simulink model "sixDOF_model3"  (R2020b)
settings: Solver=VariableStepAuto  StartTime=0.0  StopTime=Inf  RelTol=1e-3
undefined symbols (not defined in the file or in its folder): X, Y, Z
libraries: sm_lib x31, nesl_utility x31
settings Model: EnablePacing=on  PacingRate=1.100000  Creator=Idrees  LastModifiedBy=brd
settings DataIOCC: ReturnWorkspaceOutputs=off
settings DebuggingCC: ArithmeticOperatorsInVariantConditions=warning
settings SFSimCC: CustomCodeUndefinedFunction=UseInterfaceOnly

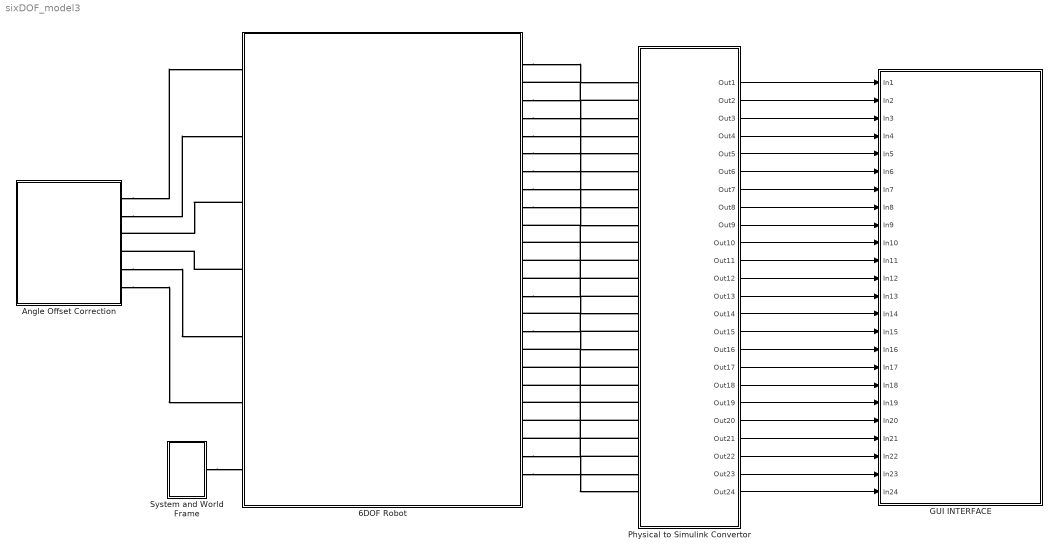
== system sixDOF_model3 ==
  6DOF Robot : Subsystem
  Angle Offset Correction : Subsystem
  GUI INTERFACE : Subsystem
  Physical to Simulink Convertor : Subsystem
  System and World Frame : Subsystem
  wires:
  Physical to Simulink Convertor/1(Out1) -> GUI INTERFACE/1(In1)
  Physical to Simulink Convertor/2(Out2) -> GUI INTERFACE/2(In2)
  Physical to Simulink Convertor/3(Out3) -> GUI INTERFACE/3(In3)
  Physical to Simulink Convertor/4(Out4) -> GUI INTERFACE/4(In4)
  Physical to Simulink Convertor/5(Out5) -> GUI INTERFACE/5(In5)
  Physical to Simulink Convertor/6(Out6) -> GUI INTERFACE/6(In6)
  Physical to Simulink Convertor/7(Out7) -> GUI INTERFACE/7(In7)
  Physical to Simulink Convertor/8(Out8) -> GUI INTERFACE/8(In8)
  Physical to Simulink Convertor/9(Out9) -> GUI INTERFACE/9(In9)
  Physical to Simulink Convertor/10(Out10) -> GUI INTERFACE/10(In10)
  Physical to Simulink Convertor/11(Out11) -> GUI INTERFACE/11(In11)
  Physical to Simulink Convertor/12(Out12) -> GUI INTERFACE/12(In12)
  Physical to Simulink Convertor/13(Out13) -> GUI INTERFACE/13(In13)
  Physical to Simulink Convertor/14(Out14) -> GUI INTERFACE/14(In14)
  Physical to Simulink Convertor/15(Out15) -> GUI INTERFACE/15(In15)
  Physical to Simulink Convertor/16(Out16) -> GUI INTERFACE/16(In16)
  Physical to Simulink Convertor/17(Out17) -> GUI INTERFACE/17(In17)
  Physical to Simulink Convertor/18(Out18) -> GUI INTERFACE/18(In18)
  Physical to Simulink Convertor/19(Out19) -> GUI INTERFACE/19(In19)
  Physical to Simulink Convertor/20(Out20) -> GUI INTERFACE/20(In20)
  Physical to Simulink Convertor/21(Out21) -> GUI INTERFACE/21(In21)
  Physical to Simulink Convertor/22(Out22) -> GUI INTERFACE/22(In22)
  Physical to Simulink Convertor/23(Out23) -> GUI INTERFACE/23(In23)
  Physical to Simulink Convertor/24(Out24) -> GUI INTERFACE/24(In24)
  connections:
  Angle Offset Correction/RConn1 -- 6DOF Robot/LConn1
  Angle Offset Correction/RConn2 -- 6DOF Robot/LConn2
  6DOF Robot/LConn3 -- Angle Offset Correction/RConn3
  6DOF Robot/LConn4 -- Angle Offset Correction/RConn4
  Angle Offset Correction/RConn5 -- 6DOF Robot/LConn5
  Angle Offset Correction/RConn6 -- 6DOF Robot/LConn6
  System and World Frame/RConn1 -- 6DOF Robot/LConn7
  6DOF Robot/RConn1 -- Physical to Simulink Convertor/LConn1
  Physical to Simulink Convertor/LConn2 -- 6DOF Robot/RConn2
  6DOF Robot/RConn3 -- Physical to Simulink Convertor/LConn3
  6DOF Robot/RConn4 -- Physical to Simulink Convertor/LConn4
  6DOF Robot/RConn5 -- Physical to Simulink Convertor/LConn5
  6DOF Robot/RConn6 -- Physical to Simulink Convertor/LConn6
  6DOF Robot/RConn7 -- Physical to Simulink Convertor/LConn7
  6DOF Robot/RConn8 -- Physical to Simulink Convertor/LConn8
  6DOF Robot/RConn9 -- Physical to Simulink Convertor/LConn9
  Physical to Simulink Convertor/LConn10 -- 6DOF Robot/RConn10
  Physical to Simulink Convertor/LConn11 -- 6DOF Robot/RConn11
  Physical to Simulink Convertor/LConn12 -- 6DOF Robot/RConn12
  Physical to Simulink Convertor/LConn13 -- 6DOF Robot/RConn13
  6DOF Robot/RConn14 -- Physical to Simulink Convertor/LConn14
  Physical to Simulink Convertor/LConn15 -- 6DOF Robot/RConn15
  6DOF Robot/RConn16 -- Physical to Simulink Convertor/LConn16
  Physical to Simulink Convertor/LConn17 -- 6DOF Robot/RConn17
  Physical to Simulink Convertor/LConn18 -- 6DOF Robot/RConn18
  Physical to Simulink Convertor/LConn19 -- 6DOF Robot/RConn19
  Physical to Simulink Convertor/LConn20 -- 6DOF Robot/RConn20
  Physical to Simulink Convertor/LConn21 -- 6DOF Robot/RConn21
  Physical to Simulink Convertor/LConn22 -- 6DOF Robot/RConn22
  6DOF Robot/RConn23 -- Physical to Simulink Convertor/LConn23
  6DOF Robot/RConn24 -- Physical to Simulink Convertor/LConn24

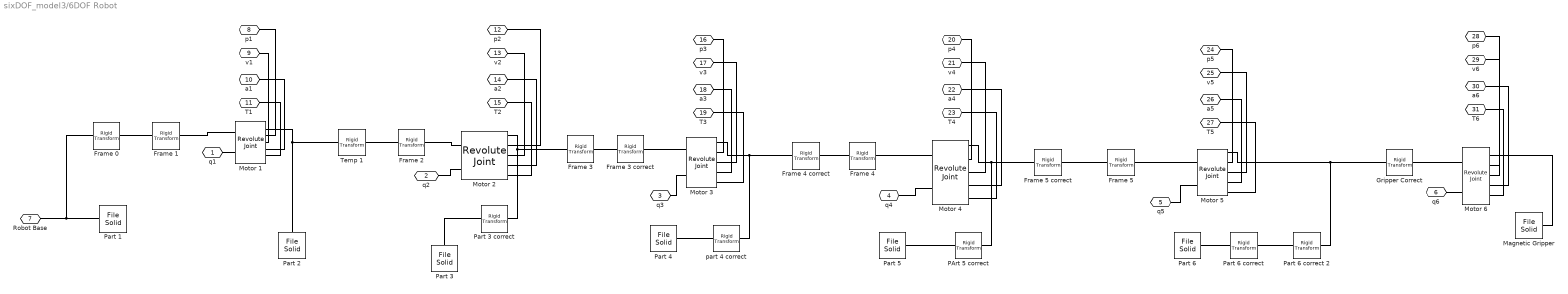
== system sixDOF_model3/6DOF Robot ==
  Frame 0 : sm_lib/Frames and Transforms/Rigid Transform  TranslationMethod=None  TranslationStandardOffset=0  TranslationLengthUnit=m  TranslationStandardAxis=+Z  TranslationCartesianOffset=[0 0 0]  TranslationROffset=0  TranslationROffsetUnits=m  TranslationZOffset=0  TranslationZOffsetUnits=m  TranslationThetaOffset=0  TranslationThetaOffsetUnits=deg  RotationMethod=StandardAxis  RotationAngleUnits=deg  RotationStandardAxis=+X  RotationAngle=90  RotationArbitraryAxis=[0 0 1]  FollAlignAxisA=+X  BaseAlignAxisA=+Y  FollAlignAxisB=+Y  BaseAlignAxisB=+Z  RotationSequenceAxes=FollowerAxes  RotationSequence=XYX  RotationSequenceAngles=[0 0 0]  RotationSequenceAnglesUnits=deg  RotationMatrix=[1 0 0; 0 1 0; 0 0 1]
  Frame 1 : sm_lib/Frames and Transforms/Rigid Transform  TranslationMethod=Cartesian  TranslationStandardOffset=60  TranslationLengthUnit=mm  TranslationStandardAxis=+Y  TranslationCartesianOffset=[0 60 0]  TranslationROffset=0  TranslationROffsetUnits=m  TranslationZOffset=0  TranslationZOffsetUnits=m  TranslationThetaOffset=0  TranslationThetaOffsetUnits=deg  RotationMethod=StandardAxis  RotationAngleUnits=deg  RotationStandardAxis=+X  RotationAngle=-90  RotationArbitraryAxis=[0 0 1]  FollAlignAxisA=+X  BaseAlignAxisA=+Y  FollAlignAxisB=+Y  BaseAlignAxisB=+Z  RotationSequenceAxes=FollowerAxes  RotationSequence=XYX  RotationSequenceAngles=[0 0 0]  RotationSequenceAnglesUnits=deg  RotationMatrix=[1 0 0; 0 1 0; 0 0 1]
  Frame 2 : sm_lib/Frames and Transforms/Rigid Transform  TranslationMethod=Cartesian  TranslationStandardOffset=0  TranslationLengthUnit=mm  TranslationStandardAxis=+Z  TranslationCartesianOffset=[0 26 29]  TranslationROffset=0  TranslationROffsetUnits=m  TranslationZOffset=0  TranslationZOffsetUnits=m  TranslationThetaOffset=0  TranslationThetaOffsetUnits=deg  RotationMethod=None  RotationAngleUnits=deg  RotationStandardAxis=+Z  RotationAngle=0.0  RotationArbitraryAxis=[0 0 1]  FollAlignAxisA=+X  BaseAlignAxisA=+Y  FollAlignAxisB=+Y  BaseAlignAxisB=+Z  RotationSequenceAxes=FollowerAxes  RotationSequence=XYX  RotationSequenceAngles=[0 0 0]  RotationSequenceAnglesUnits=deg  RotationMatrix=[1 0 0; 0 1 0; 0 0 1]
  Frame 3 : sm_lib/Frames and Transforms/Rigid Transform  TranslationMethod=Cartesian  TranslationStandardOffset=0  TranslationLengthUnit=mm  TranslationStandardAxis=+Z  TranslationCartesianOffset=[210 0 17]  TranslationROffset=0  TranslationROffsetUnits=m  TranslationZOffset=0  TranslationZOffsetUnits=m  TranslationThetaOffset=0  TranslationThetaOffsetUnits=deg  RotationMethod=StandardAxis  RotationAngleUnits=deg  RotationStandardAxis=+Z  RotationAngle=90  RotationArbitraryAxis=[0 0 1]  FollAlignAxisA=+X  BaseAlignAxisA=+Y  FollAlignAxisB=+Y  BaseAlignAxisB=+Z  RotationSequenceAxes=FollowerAxes  RotationSequence=XYX  RotationSequenceAngles=[0 0 0]  RotationSequenceAnglesUnits=deg  RotationMatrix=[1 0 0; 0 1 0; 0 0 1]
  Frame 3 correct : sm_lib/Frames and Transforms/Rigid Transform  TranslationMethod=Cartesian  TranslationStandardOffset=0  TranslationLengthUnit=mm  TranslationStandardAxis=+Z  TranslationCartesianOffset=[0 0 -60]  TranslationROffset=0  TranslationROffsetUnits=m  TranslationZOffset=0  TranslationZOffsetUnits=m  TranslationThetaOffset=0  TranslationThetaOffsetUnits=deg  RotationMethod=None  RotationAngleUnits=deg  RotationStandardAxis=+Z  RotationAngle=0.0  RotationArbitraryAxis=[0 0 1]  FollAlignAxisA=+X  BaseAlignAxisA=+Y  FollAlignAxisB=+Y  BaseAlignAxisB=+Z  RotationSequenceAxes=FollowerAxes  RotationSequence=XYX  RotationSequenceAngles=[0 0 0]  RotationSequenceAnglesUnits=deg  RotationMatrix=[1 0 0; 0 1 0; 0 0 1]
  Frame 4 : sm_lib/Frames and Transforms/Rigid Transform  TranslationMethod=Cartesian  TranslationStandardOffset=0  TranslationLengthUnit=mm  TranslationStandardAxis=+Z  TranslationCartesianOffset=[0 0 80]  TranslationROffset=0  TranslationROffsetUnits=m  TranslationZOffset=0  TranslationZOffsetUnits=m  TranslationThetaOffset=0  TranslationThetaOffsetUnits=deg  RotationMethod=StandardAxis  RotationAngleUnits=deg  RotationStandardAxis=+Z  RotationAngle=180  RotationArbitraryAxis=[0 0 1]  FollAlignAxisA=+X  BaseAlignAxisA=+Y  FollAlignAxisB=+Y  BaseAlignAxisB=+Z  RotationSequenceAxes=FollowerAxes  RotationSequence=XYX  RotationSequenceAngles=[0 0 0]  RotationSequenceAnglesUnits=deg  RotationMatrix=[1 0 0; 0 1 0; 0 0 1]
  Frame 4 correct : sm_lib/Frames and Transforms/Rigid Transform  TranslationMethod=Cartesian  TranslationStandardOffset=0  TranslationLengthUnit=mm  TranslationStandardAxis=+Z  TranslationCartesianOffset=[-180 0 0]  TranslationROffset=0  TranslationROffsetUnits=m  TranslationZOffset=0  TranslationZOffsetUnits=m  TranslationThetaOffset=0  TranslationThetaOffsetUnits=deg  RotationMethod=None  RotationAngleUnits=deg  RotationStandardAxis=+Z  RotationAngle=0.0  RotationArbitraryAxis=[0 0 1]  FollAlignAxisA=+X  BaseAlignAxisA=+Y  FollAlignAxisB=+Y  BaseAlignAxisB=+Z  RotationSequenceAxes=FollowerAxes  RotationSequence=XYX  RotationSequenceAngles=[0 0 0]  RotationSequenceAnglesUnits=deg  RotationMatrix=[1 0 0; 0 1 0; 0 0 1]
  "Frame 5 " : sm_lib/Frames and Transforms/Rigid Transform  TranslationMethod=Cartesian  TranslationStandardOffset=0  TranslationLengthUnit=mm  TranslationStandardAxis=+Z  TranslationCartesianOffset=[0 0 44.5]  TranslationROffset=0  TranslationROffsetUnits=m  TranslationZOffset=0  TranslationZOffsetUnits=m  TranslationThetaOffset=0  TranslationThetaOffsetUnits=deg  RotationMethod=None  RotationAngleUnits=deg  RotationStandardAxis=+Z  RotationAngle=0.0  RotationArbitraryAxis=[0 0 1]  FollAlignAxisA=+X  BaseAlignAxisA=+Y  FollAlignAxisB=+Y  BaseAlignAxisB=+Z  RotationSequenceAxes=FollowerAxes  RotationSequence=XYX  RotationSequenceAngles=[0 0 0]  RotationSequenceAnglesUnits=deg  RotationMatrix=[1 0 0; 0 1 0; 0 0 1]
  Frame 5 correct : sm_lib/Frames and Transforms/Rigid Transform  TranslationMethod=Cartesian  TranslationStandardOffset=0  TranslationLengthUnit=mm  TranslationStandardAxis=+Z  TranslationCartesianOffset=[0 0 21]  TranslationROffset=0  TranslationROffsetUnits=m  TranslationZOffset=0  TranslationZOffsetUnits=m  TranslationThetaOffset=0  TranslationThetaOffsetUnits=deg  RotationMethod=RotationSequence  RotationAngleUnits=deg  RotationStandardAxis=+X  RotationAngle=90  RotationArbitraryAxis=[0 0 1]  FollAlignAxisA=+X  BaseAlignAxisA=+Y  FollAlignAxisB=+Y  BaseAlignAxisB=+Z  RotationSequenceAxes=FollowerAxes  RotationSequence=XZY  RotationSequenceAngles=[90 90 0]  RotationSequenceAnglesUnits=deg  RotationMatrix=[1 0 0; 0 1 0; 0 0 1]
  Gripper Correct : sm_lib/Frames and Transforms/Rigid Transform  TranslationMethod=Cartesian  TranslationStandardOffset=0  TranslationLengthUnit=mm  TranslationStandardAxis=+Z  TranslationCartesianOffset=[-15 0 0]  TranslationROffset=0  TranslationROffsetUnits=m  TranslationZOffset=0  TranslationZOffsetUnits=m  TranslationThetaOffset=0  TranslationThetaOffsetUnits=deg  RotationMethod=StandardAxis  RotationAngleUnits=deg  RotationStandardAxis=+Y  RotationAngle=-90  RotationArbitraryAxis=[0 0 1]  FollAlignAxisA=+X  BaseAlignAxisA=+Y  FollAlignAxisB=+Y  BaseAlignAxisB=+Z  RotationSequenceAxes=FollowerAxes  RotationSequence=XYX  RotationSequenceAngles=[0 0 0]  RotationSequenceAnglesUnits=deg  RotationMatrix=[1 0 0; 0 1 0; 0 0 1]
  Magnetic Gripper : sm_lib/Body Elements/File Solid  ExtGeomFileName=/home/brd/Dropbox/School/senior-design/src/matlab/6DOF_Robot/Part7_MagneticGripper2.STEP  UnitType=FromFile  ExtGeomFileUnits=m  StepReaderType=OCC  ExportConvexHullGeometry=off  InertiaType=CalculateFromGeometry  Mass=1  MassUnits=kg  CenterOfMass=[0 0 0]  CenterOfMassUnits=m  MomentsOfInertia=[1 1 1]  MomentsOfInertiaUnits=kg*m^2  ProductsOfInertia=[0 0 0]  ProductsOfInertiaUnits=kg*m^2  BasedOnType=Density  Density=1240  DensityUnits=kg/m^3  DoExposeReferenceFrame=on  SerializedFrames=<Frames/>  GraphicType=FromGeometry  MarkerShape=Sphere  MarkerSize=10  GraphicVisPropType=SimpleVisualProperties  GraphicDiffuseColor=[0.2 0.2 0.2]  GraphicSpecularColor=[0.5 0.5 0.5 1.0]  GraphicAmbientColor=[0.15 0.15 0.15 1.0]  GraphicEmissiveColor=[0.0 0.0 0.0 1.0]  GraphicShininess=75  GraphicOpacity=1.0
  Motor {1..6} (6 alike) : sm_lib/Joints/Revolute Joint  JointMode=Normal  SenseConstraintForce=off  SenseConstraintForceX=off  SenseConstraintForceY=off  SenseConstraintForceZ=off  SenseConstraintTorque=off  SenseConstraintTorqueX=off  SenseConstraintTorqueY=off  SenseConstraintTorqueZ=off  SenseTotalForce=off  SenseTotalForceX=off  SenseTotalForceY=off  SenseTotalForceZ=off  SenseTotalTorque=off  SenseTotalTorqueX=off  SenseTotalTorqueY=off  SenseTotalTorqueZ=off  CompositeWrenchDir=FollowerOnBase  CompositeWrenchFrame=BaseFrame  EquilibriumPosition=0  EquilibriumPositionUnits=deg  SpringStiffness=0  SpringStiffnessUnits=N*m/deg  DampingCoefficient=0  DampingCoefficientUnits=N*m/(deg/s)  TorqueActuationMode=ComputedTorque  MotionActuationMode=InputMotion  SensePosition=on  SenseVelocity=on  SenseAcceleration=on  SenseTorqueForce=on  SenseLowerLimitTorqueForce=off  SenseUpperLimitTorqueForce=off  LowerLimitSpecify=off  LowerLimitBound=-90  LowerLimitBoundUnits=deg  LowerLimitStiffness=1e4  LowerLimitStiffnessUnits=N*m/deg  LowerLimitDamping=10  LowerLimitDampingUnits=N*m/(deg/s)  LowerLimitTransitionRegionWidth=0.1  LowerLimitTransitionRegionWidthUnits=deg  UpperLimitSpecify=off  UpperLimitBound=90  UpperLimitBoundUnits=deg  UpperLimitStiffness=1e4  UpperLimitStiffnessUnits=N*m/deg  UpperLimitDamping=10  UpperLimitDampingUnits=N*m/(deg/s)  UpperLimitTransitionRegionWidth=0.1  UpperLimitTransitionRegionWidthUnits=deg  PositionTargetSpecify=off  PositionTargetPriority=High  PositionTargetValue=0  PositionTargetValueUnits=deg  VelocityTargetSpecify=off  VelocityTargetPriority=High  VelocityTargetValue=0  VelocityTargetValueUnits=deg/s
  PArt 5 correct : sm_lib/Frames and Transforms/Rigid Transform  TranslationMethod=None  TranslationStandardOffset=0  TranslationLengthUnit=m  TranslationStandardAxis=+Z  TranslationCartesianOffset=[0 0 0]  TranslationROffset=0  TranslationROffsetUnits=m  TranslationZOffset=0  TranslationZOffsetUnits=m  TranslationThetaOffset=0  TranslationThetaOffsetUnits=deg  RotationMethod=StandardAxis  RotationAngleUnits=deg  RotationStandardAxis=+X  RotationAngle=180  RotationArbitraryAxis=[0 0 1]  FollAlignAxisA=+X  BaseAlignAxisA=+Y  FollAlignAxisB=+Y  BaseAlignAxisB=+Z  RotationSequenceAxes=FollowerAxes  RotationSequence=XYX  RotationSequenceAngles=[0 0 0]  RotationSequenceAnglesUnits=deg  RotationMatrix=[1 0 0; 0 1 0; 0 0 1]
  "Part 1 " : sm_lib/Body Elements/File Solid  ExtGeomFileName=/home/brd/Dropbox/School/senior-design/src/matlab/6DOF_Robot/Part1.STEP  UnitType=FromFile  ExtGeomFileUnits=m  StepReaderType=OCC  ExportConvexHullGeometry=off  InertiaType=CalculateFromGeometry  Mass=1  MassUnits=kg  CenterOfMass=[0 0 0]  CenterOfMassUnits=m  MomentsOfInertia=[1 1 1]  MomentsOfInertiaUnits=kg*m^2  ProductsOfInertia=[0 0 0]  ProductsOfInertiaUnits=kg*m^2  BasedOnType=Density  Density=1240  DensityUnits=kg/m^3  DoExposeReferenceFrame=on  SerializedFrames=<Frames/>  GraphicType=FromGeometry  MarkerShape=Sphere  MarkerSize=10  GraphicVisPropType=SimpleVisualProperties  GraphicDiffuseColor=[1.0 0.6 0.2]  GraphicSpecularColor=[0.5 0.5 0.5 1.0]  GraphicAmbientColor=[0.15 0.15 0.15 1.0]  GraphicEmissiveColor=[0.0 0.0 0.0 1.0]  GraphicShininess=75  GraphicOpacity=1.0
  Part 2 : sm_lib/Body Elements/File Solid  ExtGeomFileName=/home/brd/Dropbox/School/senior-design/src/matlab/6DOF_Robot/Part2.STEP  UnitType=FromFile  ExtGeomFileUnits=m  StepReaderType=OCC  ExportConvexHullGeometry=off  InertiaType=CalculateFromGeometry  Mass=1  MassUnits=kg  CenterOfMass=[0 0 0]  CenterOfMassUnits=m  MomentsOfInertia=[1 1 1]  MomentsOfInertiaUnits=kg*m^2  ProductsOfInertia=[0 0 0]  ProductsOfInertiaUnits=kg*m^2  BasedOnType=Density  Density=1240  DensityUnits=kg/m^3  DoExposeReferenceFrame=on  SerializedFrames=<Frames/>  GraphicType=FromGeometry  MarkerShape=Sphere  MarkerSize=10  GraphicVisPropType=SimpleVisualProperties  GraphicDiffuseColor=[1.0 0.4 0.0]  GraphicSpecularColor=[0.5 0.5 0.5 1.0]  GraphicAmbientColor=[0.15 0.15 0.15 1.0]  GraphicEmissiveColor=[0.0 0.0 0.0 1.0]  GraphicShininess=75  GraphicOpacity=1.0
  Part 3 : sm_lib/Body Elements/File Solid  ExtGeomFileName=/home/brd/Dropbox/School/senior-design/src/matlab/6DOF_Robot/Part3.STEP  UnitType=FromFile  ExtGeomFileUnits=m  StepReaderType=OCC  ExportConvexHullGeometry=off  InertiaType=CalculateFromGeometry  Mass=1  MassUnits=kg  CenterOfMass=[0 0 0]  CenterOfMassUnits=m  MomentsOfInertia=[1 1 1]  MomentsOfInertiaUnits=kg*m^2  ProductsOfInertia=[0 0 0]  ProductsOfInertiaUnits=kg*m^2  BasedOnType=Density  Density=1240  DensityUnits=kg/m^3  DoExposeReferenceFrame=on  SerializedFrames=<Frames/>  GraphicType=FromGeometry  MarkerShape=Sphere  MarkerSize=10  GraphicVisPropType=SimpleVisualProperties  GraphicDiffuseColor=[1.0 0.4 0.0]  GraphicSpecularColor=[0.5 0.5 0.5 1.0]  GraphicAmbientColor=[0.15 0.15 0.15 1.0]  GraphicEmissiveColor=[0.0 0.0 0.0 1.0]  GraphicShininess=75  GraphicOpacity=1.0
  Part 3 correct : sm_lib/Frames and Transforms/Rigid Transform  TranslationMethod=Cartesian  TranslationStandardOffset=0  TranslationLengthUnit=mm  TranslationStandardAxis=+Z  TranslationCartesianOffset=[-210/2 0 0]  TranslationROffset=0  TranslationROffsetUnits=m  TranslationZOffset=0  TranslationZOffsetUnits=m  TranslationThetaOffset=0  TranslationThetaOffsetUnits=deg  RotationMethod=None  RotationAngleUnits=deg  RotationStandardAxis=+Z  RotationAngle=0.0  RotationArbitraryAxis=[0 0 1]  FollAlignAxisA=+X  BaseAlignAxisA=+Y  FollAlignAxisB=+Y  BaseAlignAxisB=+Z  RotationSequenceAxes=FollowerAxes  RotationSequence=XYX  RotationSequenceAngles=[0 0 0]  RotationSequenceAnglesUnits=deg  RotationMatrix=[1 0 0; 0 1 0; 0 0 1]
  Part 4 : sm_lib/Body Elements/File Solid  ExtGeomFileName=/home/brd/Dropbox/School/senior-design/src/matlab/6DOF_Robot/Part4.STEP  UnitType=FromFile  ExtGeomFileUnits=m  StepReaderType=OCC  ExportConvexHullGeometry=off  InertiaType=CalculateFromGeometry  Mass=1  MassUnits=kg  CenterOfMass=[0 0 0]  CenterOfMassUnits=m  MomentsOfInertia=[1 1 1]  MomentsOfInertiaUnits=kg*m^2  ProductsOfInertia=[0 0 0]  ProductsOfInertiaUnits=kg*m^2  BasedOnType=Density  Density=1240  DensityUnits=kg/m^3  DoExposeReferenceFrame=on  SerializedFrames=<Frames/>  GraphicType=FromGeometry  MarkerShape=Sphere  MarkerSize=10  GraphicVisPropType=SimpleVisualProperties  GraphicDiffuseColor=[1.0 0.4 0.0]  GraphicSpecularColor=[0.5 0.5 0.5 1.0]  GraphicAmbientColor=[0.15 0.15 0.15 1.0]  GraphicEmissiveColor=[0.0 0.0 0.0 1.0]  GraphicShininess=75  GraphicOpacity=1.0
  Part 5 : sm_lib/Body Elements/File Solid  ExtGeomFileName=/home/brd/Dropbox/School/senior-design/src/matlab/6DOF_Robot/Part5.STEP  UnitType=FromFile  ExtGeomFileUnits=m  StepReaderType=OCC  ExportConvexHullGeometry=off  InertiaType=CalculateFromGeometry  Mass=1  MassUnits=kg  CenterOfMass=[0 0 0]  CenterOfMassUnits=m  MomentsOfInertia=[1 1 1]  MomentsOfInertiaUnits=kg*m^2  ProductsOfInertia=[0 0 0]  ProductsOfInertiaUnits=kg*m^2  BasedOnType=Density  Density=1240  DensityUnits=kg/m^3  DoExposeReferenceFrame=on  SerializedFrames=<Frames/>  GraphicType=FromGeometry  MarkerShape=Sphere  MarkerSize=10  GraphicVisPropType=SimpleVisualProperties  GraphicDiffuseColor=[1.0 0.4 0.0]  GraphicSpecularColor=[0.5 0.5 0.5 1.0]  GraphicAmbientColor=[0.15 0.15 0.15 1.0]  GraphicEmissiveColor=[0.0 0.0 0.0 1.0]  GraphicShininess=75  GraphicOpacity=1.0
  Part 6 : sm_lib/Body Elements/File Solid  ExtGeomFileName=/home/brd/Dropbox/School/senior-design/src/matlab/6DOF_Robot/Part6.STEP  UnitType=FromFile  ExtGeomFileUnits=m  StepReaderType=OCC  ExportConvexHullGeometry=off  InertiaType=CalculateFromGeometry  Mass=1  MassUnits=kg  CenterOfMass=[0 0 0]  CenterOfMassUnits=m  MomentsOfInertia=[1 1 1]  MomentsOfInertiaUnits=kg*m^2  ProductsOfInertia=[0 0 0]  ProductsOfInertiaUnits=kg*m^2  BasedOnType=Density  Density=1240  DensityUnits=kg/m^3  DoExposeReferenceFrame=on  SerializedFrames=<Frames/>  GraphicType=FromGeometry  MarkerShape=Sphere  MarkerSize=10  GraphicVisPropType=SimpleVisualProperties  GraphicDiffuseColor=[1.0 0.4 0.0]  GraphicSpecularColor=[0.5 0.5 0.5 1.0]  GraphicAmbientColor=[0.15 0.15 0.15 1.0]  GraphicEmissiveColor=[0.0 0.0 0.0 1.0]  GraphicShininess=75  GraphicOpacity=1.0
  Part 6 correct : sm_lib/Frames and Transforms/Rigid Transform  TranslationMethod=Cartesian  TranslationStandardOffset=0  TranslationLengthUnit=mm  TranslationStandardAxis=+Z  TranslationCartesianOffset=[0 0 15]  TranslationROffset=0  TranslationROffsetUnits=m  TranslationZOffset=0  TranslationZOffsetUnits=m  TranslationThetaOffset=0  TranslationThetaOffsetUnits=deg  RotationMethod=None  RotationAngleUnits=deg  RotationStandardAxis=+X  RotationAngle=90  RotationArbitraryAxis=[0 0 1]  FollAlignAxisA=+X  BaseAlignAxisA=+Y  FollAlignAxisB=+Y  BaseAlignAxisB=+Z  RotationSequenceAxes=FollowerAxes  RotationSequence=XYX  RotationSequenceAngles=[0 0 0]  RotationSequenceAnglesUnits=deg  RotationMatrix=[1 0 0; 0 1 0; 0 0 1]
  Part 6 correct 2 : sm_lib/Frames and Transforms/Rigid Transform  TranslationMethod=None  TranslationStandardOffset=0  TranslationLengthUnit=m  TranslationStandardAxis=+Z  TranslationCartesianOffset=[0 0 0]  TranslationROffset=0  TranslationROffsetUnits=m  TranslationZOffset=0  TranslationZOffsetUnits=m  TranslationThetaOffset=0  TranslationThetaOffsetUnits=deg  RotationMethod=RotationSequence  RotationAngleUnits=deg  RotationStandardAxis=+Z  RotationAngle=0.0  RotationArbitraryAxis=[0 0 1]  FollAlignAxisA=+X  BaseAlignAxisA=+Y  FollAlignAxisB=+Y  BaseAlignAxisB=+Z  RotationSequenceAxes=FollowerAxes  RotationSequence=ZYX  RotationSequenceAngles=[90 -90 0]  RotationSequenceAnglesUnits=deg  RotationMatrix=[1 0 0; 0 1 0; 0 0 1]
  Temp 1 : sm_lib/Frames and Transforms/Rigid Transform  TranslationMethod=None  TranslationStandardOffset=0  TranslationLengthUnit=m  TranslationStandardAxis=+Z  TranslationCartesianOffset=[0 0 0]  TranslationROffset=0  TranslationROffsetUnits=m  TranslationZOffset=0  TranslationZOffsetUnits=m  TranslationThetaOffset=0  TranslationThetaOffsetUnits=deg  RotationMethod=StandardAxis  RotationAngleUnits=deg  RotationStandardAxis=+X  RotationAngle=90  RotationArbitraryAxis=[0 0 1]  FollAlignAxisA=+X  BaseAlignAxisA=+Y  FollAlignAxisB=+Y  BaseAlignAxisB=+Z  RotationSequenceAxes=FollowerAxes  RotationSequence=XYX  RotationSequenceAngles=[0 0 0]  RotationSequenceAnglesUnits=deg  RotationMatrix=[1 0 0; 0 1 0; 0 0 1]
  part 4 correct : sm_lib/Frames and Transforms/Rigid Transform  TranslationMethod=Cartesian  TranslationStandardOffset=0  TranslationLengthUnit=mm  TranslationStandardAxis=+Z  TranslationCartesianOffset=[180/2 0 0]  TranslationROffset=0  TranslationROffsetUnits=m  TranslationZOffset=0  TranslationZOffsetUnits=m  TranslationThetaOffset=0  TranslationThetaOffsetUnits=deg  RotationMethod=None  RotationAngleUnits=deg  RotationStandardAxis=+Z  RotationAngle=0.0  RotationArbitraryAxis=[0 0 1]  FollAlignAxisA=+X  BaseAlignAxisA=+Y  FollAlignAxisB=+Y  BaseAlignAxisB=+Z  RotationSequenceAxes=FollowerAxes  RotationSequence=XYX  RotationSequenceAngles=[0 0 0]  RotationSequenceAnglesUnits=deg  RotationMatrix=[1 0 0; 0 1 0; 0 0 1]
  q1 : PMIOPort  Side=Left
  q2 : PMIOPort  Port=2  Side=Left
  q3 : PMIOPort  Port=3  Side=Left
  q4 : PMIOPort  Port=4  Side=Left
  q5 : PMIOPort  Port=5  Side=Left
  q6 : PMIOPort  Port=6  Side=Left
  Robot Base : PMIOPort  Port=7  Side=Left
  p1 : PMIOPort  Port=8  Side=Right
  v1 : PMIOPort  Port=9  Side=Right
  a1 : PMIOPort  Port=10  Side=Right
  T1 : PMIOPort  Port=11  Side=Right
  p2 : PMIOPort  Port=12  Side=Right
  v2 : PMIOPort  Port=13  Side=Right
  a2 : PMIOPort  Port=14  Side=Right
  T2 : PMIOPort  Port=15  Side=Right
  p3 : PMIOPort  Port=16  Side=Right
  v3 : PMIOPort  Port=17  Side=Right
  a3 : PMIOPort  Port=18  Side=Right
  T3 : PMIOPort  Port=19  Side=Right
  p4 : PMIOPort  Port=20  Side=Right
  v4 : PMIOPort  Port=21  Side=Right
  a4 : PMIOPort  Port=22  Side=Right
  T4 : PMIOPort  Port=23  Side=Right
  p5 : PMIOPort  Port=24  Side=Right
  v5 : PMIOPort  Port=25  Side=Right
  a5 : PMIOPort  Port=26  Side=Right
  T5 : PMIOPort  Port=27  Side=Right
  p6 : PMIOPort  Port=28  Side=Right
  v6 : PMIOPort  Port=29  Side=Right
  a6 : PMIOPort  Port=30  Side=Right
  T6 : PMIOPort  Port=31  Side=Right
  connections:
  Motor 1/LConn1 -- Frame 1/RConn1
  Motor 4/RConn1 -- Frame 5 correct/LConn1 -- PArt 5 correct/RConn1
  part 4 correct/RConn1 -- Motor 3/RConn1 -- Frame 4 correct/LConn1
  Frame 1/LConn1 -- Frame 0/RConn1
  Part 6 correct/LConn1 -- Part 6/RConn1
  part 4 correct/LConn1 -- Part 4/RConn1
  Magnetic Gripper/RConn1 -- Motor 6/RConn1
  Frame 4/LConn1 -- Frame 4 correct/RConn1
  "Part 1 "/RConn1 -- Robot Base/RConn1 -- Frame 0/LConn1
  Motor 1/RConn1 -- Temp 1/LConn1 -- Part 2/RConn1
  Part 6 correct 2/RConn1 -- Motor 5/RConn1 -- Gripper Correct/LConn1
  Motor 6/LConn1 -- Gripper Correct/RConn1
  Frame 3 correct/LConn1 -- Frame 3/RConn1
  Temp 1/RConn1 -- Frame 2/LConn1
  Motor 3/LConn1 -- Frame 3 correct/RConn1
  Motor 2/LConn2 -- q2/RConn1
  "Frame 5 "/LConn1 -- Frame 5 correct/RConn1
  Motor 2/RConn1 -- Part 3 correct/RConn1 -- Frame 3/LConn1
  Motor 2/LConn1 -- Frame 2/RConn1
  Part 3 correct/LConn1 -- Part 3/RConn1
  Frame 4/RConn1 -- Motor 4/LConn1
  Motor 5/LConn1 -- "Frame 5 "/RConn1
  PArt 5 correct/LConn1 -- Part 5/RConn1
  Part 6 correct 2/LConn1 -- Part 6 correct/RConn1
  Motor 1/LConn2 -- q1/RConn1
  Motor 3/LConn2 -- q3/RConn1
  Motor 4/LConn2 -- q4/RConn1
  Motor 5/LConn2 -- q5/RConn1
  q6/RConn1 -- Motor 6/LConn2
  T2/RConn1 -- Motor 2/RConn5
  p2/RConn1 -- Motor 2/RConn2
  v2/RConn1 -- Motor 2/RConn3
  a2/RConn1 -- Motor 2/RConn4
  p1/RConn1 -- Motor 1/RConn2
  v1/RConn1 -- Motor 1/RConn3
  a1/RConn1 -- Motor 1/RConn4
  T1/RConn1 -- Motor 1/RConn5
  p3/RConn1 -- Motor 3/RConn2
  v3/RConn1 -- Motor 3/RConn3
  a3/RConn1 -- Motor 3/RConn4
  T3/RConn1 -- Motor 3/RConn5
  p4/RConn1 -- Motor 4/RConn2
  v4/RConn1 -- Motor 4/RConn3
  a4/RConn1 -- Motor 4/RConn4
  T4/RConn1 -- Motor 4/RConn5
  p5/RConn1 -- Motor 5/RConn2
  v5/RConn1 -- Motor 5/RConn3
  a5/RConn1 -- Motor 5/RConn4
  T5/RConn1 -- Motor 5/RConn5
  p6/RConn1 -- Motor 6/RConn2
  v6/RConn1 -- Motor 6/RConn3
  a6/RConn1 -- Motor 6/RConn4
  T6/RConn1 -- Motor 6/RConn5

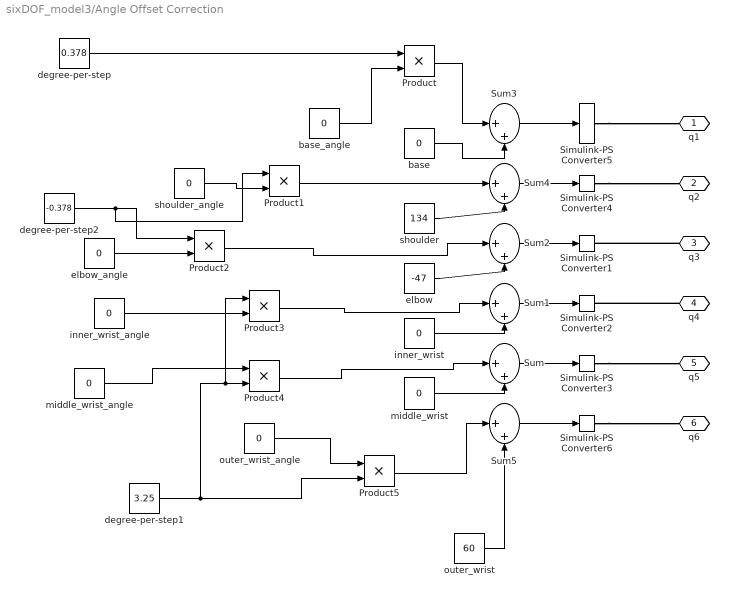
== system sixDOF_model3/Angle Offset Correction ==
  Product{,1..5} (6 alike) : Product
  Simulink-PS Converter{1..4,6} (5 alike) : nesl_utility/Simulink-PS Converter  PhysicalDomain=network_engine_domain  SubClassName=ps_input  LeftPortType=input  RightPortType=output  PseudoPeriodic=off  Frequencies=[]  NoiseDistribution=none  NoiseParameters=[]  Unit=deg  AffineConversion=off  FilteringAndDerivatives=filter  SimscapeFilterOrder=2  InputFilterTimeConstant=0.001  UdotUserProvided=0
  Simulink-PS Converter5 : nesl_utility/Simulink-PS Converter  PhysicalDomain=network_engine_domain  SubClassName=ps_input  LeftPortType=input  RightPortType=output  PseudoPeriodic=off  Frequencies=[]  NoiseDistribution=none  NoiseParameters=[]  Unit=deg  AffineConversion=off  FilteringAndDerivatives=filter  SimscapeFilterOrder=2  InputFilterTimeConstant=0.001  UdotUserProvided=2
  Sum{,1..5} (6 alike) : Sum  Inputs=|++
  base : Constant  Value=0
  base_angle : Constant  Value=0  VectorParams1D=off
  degree-per-step : Constant  Value=0.378  VectorParams1D=off
  degree-per-step1 : Constant  Value=3.25  VectorParams1D=off
  degree-per-step2 : Constant  Value=-0.378  VectorParams1D=off
  elbow : Constant  Value=-47
  elbow_angle : Constant  Value=0
  inner_wrist : Constant  Value=0
  inner_wrist_angle : Constant  Value=0
  middle_wrist : Constant  Value=0
  middle_wrist_angle : Constant  Value=0
  outer_wrist : Constant  Value=60
  outer_wrist_angle : Constant  Value=0
  shoulder : Constant  Value=134
  shoulder_angle : Constant  Value=0
  q1 : PMIOPort  Side=Right
  q2 : PMIOPort  Port=2  Side=Right
  q3 : PMIOPort  Port=3  Side=Right
  q4 : PMIOPort  Port=4  Side=Right
  q5 : PMIOPort  Port=5  Side=Right
  q6 : PMIOPort  Port=6  Side=Right
  wires:
  elbow/1 -> Sum2/2
  middle_wrist/1 -> Sum/2
  Sum/1 -> Simulink-PS Converter3/1
  inner_wrist/1 -> Sum1/2
  Sum2/1 -> Simulink-PS Converter1/1
  Sum1/1 -> Simulink-PS Converter2/1
  shoulder/1 -> Sum4/2
  Sum4/1 -> Simulink-PS Converter4/1
  Sum3/1 -> Simulink-PS Converter5/1
  outer_wrist/1 -> Sum5/2
  Sum5/1 -> Simulink-PS Converter6/1
  base_angle/1 -> Product/2
  Product/1 -> Sum3/1
  base/1 -> Sum3/2
  degree-per-step/1 -> Product/1
  outer_wrist_angle/1 -> Product5/1
  degree-per-step1/1 -> Product3/1, Product4/2, Product5/2
  Product5/1 -> Sum5/1
  middle_wrist_angle/1 -> Product4/1
  Product4/1 -> Sum/1
  inner_wrist_angle/1 -> Product3/2
  Product3/1 -> Sum1/1
  elbow_angle/1 -> Product2/2
  Product2/1 -> Sum2/1
  shoulder_angle/1 -> Product1/2
  Product1/1 -> Sum4/1
  degree-per-step2/1 -> Product1/1, Product2/1
  connections:
  q3/RConn1 -- Simulink-PS Converter1/RConn1
  Simulink-PS Converter4/RConn1 -- q2/RConn1
  q4/RConn1 -- Simulink-PS Converter2/RConn1
  Simulink-PS Converter5/RConn1 -- q1/RConn1
  Simulink-PS Converter3/RConn1 -- q5/RConn1
  Simulink-PS Converter6/RConn1 -- q6/RConn1

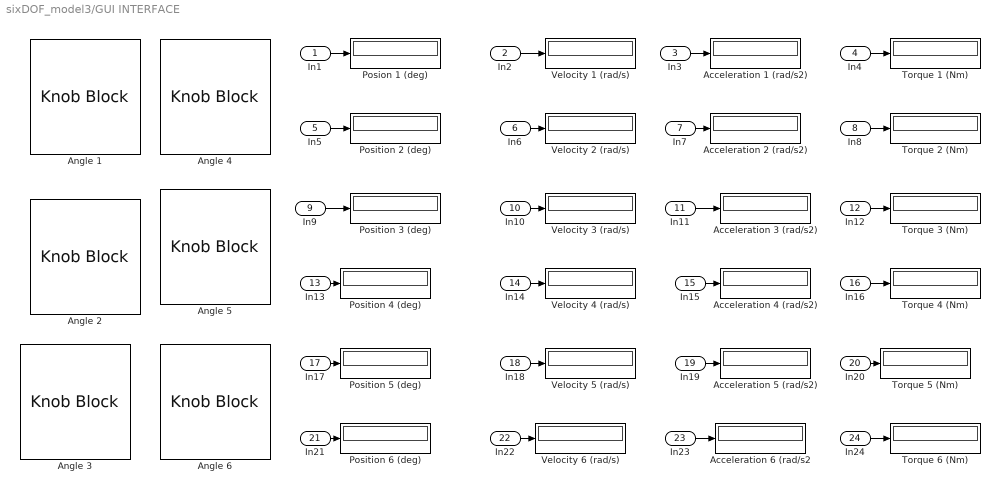
== system sixDOF_model3/GUI INTERFACE ==
  In1 : Inport
  In2 : Inport  Port=2
  In3 : Inport  Port=3
  In4 : Inport  Port=4
  In5 : Inport  Port=5
  In6 : Inport  Port=6
  In7 : Inport  Port=7
  In8 : Inport  Port=8
  In9 : Inport  Port=9
  In10 : Inport  Port=10
  In11 : Inport  Port=11
  In12 : Inport  Port=12
  In13 : Inport  Port=13
  In14 : Inport  Port=14
  In15 : Inport  Port=15
  In16 : Inport  Port=16
  In17 : Inport  Port=17
  In18 : Inport  Port=18
  In19 : Inport  Port=19
  In20 : Inport  Port=20
  In21 : Inport  Port=21
  In22 : Inport  Port=22
  In23 : Inport  Port=23
  In24 : Inport  Port=24
  Acceleration 1 (rad/s2) : Display
  Acceleration 2 (rad/s2) : Display
  Acceleration 3 (rad/s2) : Display
  Acceleration 4 (rad/s2) : Display
  Acceleration 5 (rad/s2) : Display
  Acceleration 6 (rad/s2 : Display
  Angle {1..6} (6 alike) : KnobBlock  ScaleMin=-180  ScaleMax=180
  "Posion 1 (deg) " : Display
  "Position 2 (deg) " : Display
  "Position 3 (deg) " : Display
  "Position 4 (deg) " : Display
  "Position 5 (deg) " : Display
  "Position 6 (deg) " : Display
  Torque 1 (Nm) : Display
  Torque 2 (Nm) : Display
  Torque 3 (Nm) : Display
  Torque 4 (Nm) : Display
  Torque 5 (Nm) : Display
  Torque 6 (Nm) : Display
  Velocity 1 (rad/s) : Display
  Velocity 2 (rad/s) : Display
  Velocity 3 (rad/s) : Display
  Velocity 4 (rad/s) : Display
  Velocity 5 (rad/s) : Display
  Velocity 6 (rad/s) : Display
  wires:
  In1/1 -> "Posion 1 (deg) "/1
  In6/1 -> Velocity 2 (rad/s)/1
  In10/1 -> Velocity 3 (rad/s)/1
  In3/1 -> Acceleration 1 (rad/s2)/1
  In8/1 -> Torque 2 (Nm)/1
  In5/1 -> "Position 2 (deg) "/1
  In4/1 -> Torque 1 (Nm)/1
  In9/1 -> "Position 3 (deg) "/1
  In2/1 -> Velocity 1 (rad/s)/1
  In7/1 -> Acceleration 2 (rad/s2)/1
  In12/1 -> Torque 3 (Nm)/1
  In17/1 -> "Position 5 (deg) "/1
  In11/1 -> Acceleration 3 (rad/s2)/1
  In15/1 -> Acceleration 4 (rad/s2)/1
  In13/1 -> "Position 4 (deg) "/1
  In14/1 -> Velocity 4 (rad/s)/1
  In16/1 -> Torque 4 (Nm)/1
  In19/1 -> Acceleration 5 (rad/s2)/1
  In18/1 -> Velocity 5 (rad/s)/1
  In20/1 -> Torque 5 (Nm)/1
  In21/1 -> "Position 6 (deg) "/1
  In22/1 -> Velocity 6 (rad/s)/1
  In23/1 -> Acceleration 6 (rad/s2/1
  In24/1 -> Torque 6 (Nm)/1

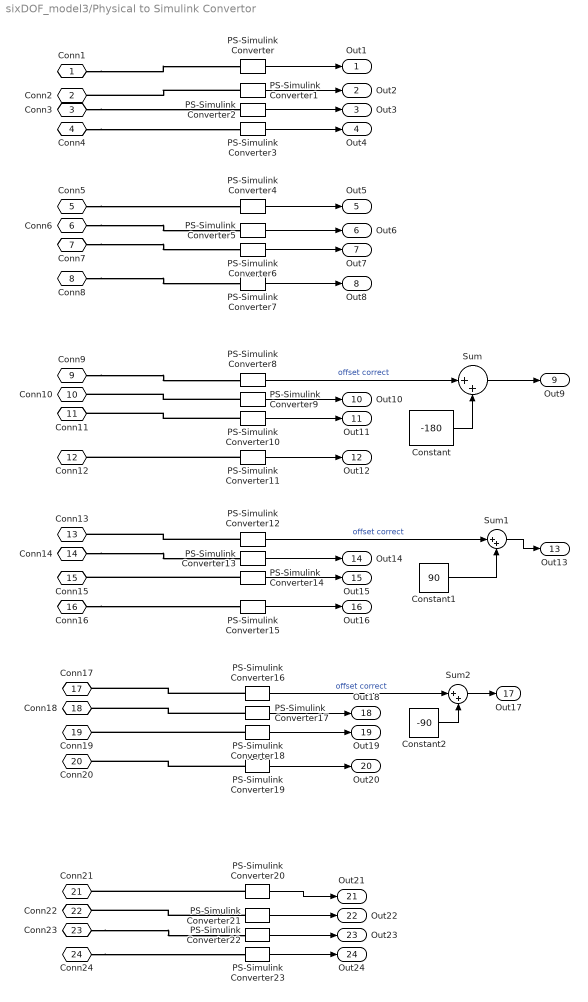
== system sixDOF_model3/Physical to Simulink Convertor ==
  Constant : Constant  Value=-180
  Constant1 : Constant  Value=90
  Constant2 : Constant  Value=-90
  PS-Simulink Converter{,4,8,12,16,20} (6 alike) : nesl_utility/PS-Simulink Converter  PhysicalDomain=network_engine_domain  SubClassName=ps_output  LeftPortType=input  RightPortType=output  PseudoPeriodic=off  Frequencies=[]  Unit=deg  AffineConversion=off
  PS-Simulink Converter{1,5,9,13,17,21} (6 alike) : nesl_utility/PS-Simulink Converter  PhysicalDomain=network_engine_domain  SubClassName=ps_output  LeftPortType=input  RightPortType=output  PseudoPeriodic=off  Frequencies=[]  Unit=rad/s  AffineConversion=off
  PS-Simulink Converter{2,6,10,14,18,22} (6 alike) : nesl_utility/PS-Simulink Converter  PhysicalDomain=network_engine_domain  SubClassName=ps_output  LeftPortType=input  RightPortType=output  PseudoPeriodic=off  Frequencies=[]  Unit=rad/s^2  AffineConversion=off
  PS-Simulink Converter{3,7,11,15,19,23} (6 alike) : nesl_utility/PS-Simulink Converter  PhysicalDomain=network_engine_domain  SubClassName=ps_output  LeftPortType=input  RightPortType=output  PseudoPeriodic=off  Frequencies=[]  Unit=N*m  AffineConversion=off
  Sum : Sum  Inputs=|++
  Sum1 : Sum  Inputs=|++
  Sum2 : Sum  Inputs=|++
  Conn1 : PMIOPort  Side=Left
  Conn2 : PMIOPort  Port=2  Side=Left
  Conn3 : PMIOPort  Port=3  Side=Left
  Conn4 : PMIOPort  Port=4  Side=Left
  Conn5 : PMIOPort  Port=5  Side=Left
  Conn6 : PMIOPort  Port=6  Side=Left
  Conn7 : PMIOPort  Port=7  Side=Left
  Conn8 : PMIOPort  Port=8  Side=Left
  Conn9 : PMIOPort  Port=9  Side=Left
  Conn10 : PMIOPort  Port=10  Side=Left
  Conn11 : PMIOPort  Port=11  Side=Left
  Conn12 : PMIOPort  Port=12  Side=Left
  Conn13 : PMIOPort  Port=13  Side=Left
  Conn14 : PMIOPort  Port=14  Side=Left
  Conn15 : PMIOPort  Port=15  Side=Left
  Conn16 : PMIOPort  Port=16  Side=Left
  Conn17 : PMIOPort  Port=17  Side=Left
  Conn18 : PMIOPort  Port=18  Side=Left
  Conn19 : PMIOPort  Port=19  Side=Left
  Conn20 : PMIOPort  Port=20  Side=Left
  Conn21 : PMIOPort  Port=21  Side=Left
  Conn22 : PMIOPort  Port=22  Side=Left
  Conn23 : PMIOPort  Port=23  Side=Left
  Conn24 : PMIOPort  Port=24  Side=Left
  Out1 : Outport  VectorParamsAs1DForOutWhenUnconnected=off
  Out2 : Outport  Port=2  VectorParamsAs1DForOutWhenUnconnected=off
  Out3 : Outport  Port=3  VectorParamsAs1DForOutWhenUnconnected=off
  Out4 : Outport  Port=4  VectorParamsAs1DForOutWhenUnconnected=off
  Out5 : Outport  Port=5  VectorParamsAs1DForOutWhenUnconnected=off
  Out6 : Outport  Port=6  VectorParamsAs1DForOutWhenUnconnected=off
  Out7 : Outport  Port=7  VectorParamsAs1DForOutWhenUnconnected=off
  Out8 : Outport  Port=8  VectorParamsAs1DForOutWhenUnconnected=off
  Out9 : Outport  Port=9  VectorParamsAs1DForOutWhenUnconnected=off
  Out10 : Outport  Port=10  VectorParamsAs1DForOutWhenUnconnected=off
  Out11 : Outport  Port=11  VectorParamsAs1DForOutWhenUnconnected=off
  Out12 : Outport  Port=12  VectorParamsAs1DForOutWhenUnconnected=off
  Out13 : Outport  Port=13  VectorParamsAs1DForOutWhenUnconnected=off
  Out14 : Outport  Port=14  VectorParamsAs1DForOutWhenUnconnected=off
  Out15 : Outport  Port=15  VectorParamsAs1DForOutWhenUnconnected=off
  Out16 : Outport  Port=16  VectorParamsAs1DForOutWhenUnconnected=off
  Out17 : Outport  Port=17  VectorParamsAs1DForOutWhenUnconnected=off
  Out18 : Outport  Port=18  VectorParamsAs1DForOutWhenUnconnected=off
  Out19 : Outport  Port=19  VectorParamsAs1DForOutWhenUnconnected=off
  Out20 : Outport  Port=20  VectorParamsAs1DForOutWhenUnconnected=off
  Out21 : Outport  Port=21  VectorParamsAs1DForOutWhenUnconnected=off
  Out22 : Outport  Port=22  VectorParamsAs1DForOutWhenUnconnected=off
  Out23 : Outport  Port=23  VectorParamsAs1DForOutWhenUnconnected=off
  Out24 : Outport  Port=24  VectorParamsAs1DForOutWhenUnconnected=off
  wires:
  PS-Simulink Converter15/1 -> Out16/1
  PS-Simulink Converter6/1 -> Out7/1
  PS-Simulink Converter13/1 -> Out14/1
  PS-Simulink Converter23/1 -> Out24/1
  PS-Simulink Converter2/1 -> Out3/1
  PS-Simulink Converter4/1 -> Out5/1
  PS-Simulink Converter10/1 -> Out11/1
  PS-Simulink Converter/1 -> Out1/1
  PS-Simulink Converter9/1 -> Out10/1
  PS-Simulink Converter7/1 -> Out8/1
  PS-Simulink Converter17/1 -> Out18/1
  PS-Simulink Converter20/1 -> Out21/1
  PS-Simulink Converter3/1 -> Out4/1
  PS-Simulink Converter22/1 -> Out23/1
  PS-Simulink Converter14/1 -> Out15/1
  PS-Simulink Converter5/1 -> Out6/1
  PS-Simulink Converter1/1 -> Out2/1
  PS-Simulink Converter19/1 -> Out20/1
  PS-Simulink Converter21/1 -> Out22/1
  PS-Simulink Converter11/1 -> Out12/1
  PS-Simulink Converter18/1 -> Out19/1
  Constant/1 -> Sum/2
  PS-Simulink Converter8/1 -> Sum/1  "offset correct"
  Sum/1 -> Out9/1
  Constant1/1 -> Sum1/2
  PS-Simulink Converter12/1 -> Sum1/1  "offset correct"
  Sum1/1 -> Out13/1
  Constant2/1 -> Sum2/2
  PS-Simulink Converter16/1 -> Sum2/1  "offset correct"
  Sum2/1 -> Out17/1
  connections:
  PS-Simulink Converter14/LConn1 -- Conn15/RConn1
  Conn14/RConn1 -- PS-Simulink Converter13/LConn1
  PS-Simulink Converter16/LConn1 -- Conn17/RConn1
  Conn4/RConn1 -- PS-Simulink Converter3/LConn1
  Conn23/RConn1 -- PS-Simulink Converter22/LConn1
  PS-Simulink Converter12/LConn1 -- Conn13/RConn1
  Conn8/RConn1 -- PS-Simulink Converter7/LConn1
  PS-Simulink Converter18/LConn1 -- Conn19/RConn1
  Conn24/RConn1 -- PS-Simulink Converter23/LConn1
  PS-Simulink Converter17/LConn1 -- Conn18/RConn1
  PS-Simulink Converter9/LConn1 -- Conn10/RConn1
  PS-Simulink Converter10/LConn1 -- Conn11/RConn1
  Conn6/RConn1 -- PS-Simulink Converter5/LConn1
  Conn16/RConn1 -- PS-Simulink Converter15/LConn1
  Conn9/RConn1 -- PS-Simulink Converter8/LConn1
  Conn1/RConn1 -- PS-Simulink Converter/LConn1
  PS-Simulink Converter21/LConn1 -- Conn22/RConn1
  Conn7/RConn1 -- PS-Simulink Converter6/LConn1
  PS-Simulink Converter11/LConn1 -- Conn12/RConn1
  PS-Simulink Converter20/LConn1 -- Conn21/RConn1
  PS-Simulink Converter19/LConn1 -- Conn20/RConn1
  PS-Simulink Converter1/LConn1 -- Conn2/RConn1
  Conn5/RConn1 -- PS-Simulink Converter4/LConn1
  Conn3/RConn1 -- PS-Simulink Converter2/LConn1

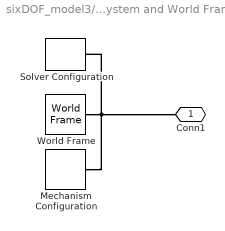
== system sixDOF_model3/System and World Frame ==
  Mechanism Configuration : sm_lib/Utilities/Mechanism Configuration  UniformGravity=Constant  GravityVector=[0 0 -9.81]  GravityVectorUnits=m/s^2  GravityUnits=m/s^2  LinearizationDelta=0.001  JointModeTransitionNonlinearIterations=2
  Solver Configuration : nesl_utility/Solver Configuration  PhysicalDomain=network_engine_domain  SubClassName=solver  LeftPortType=input  RightPortType=generic  Tones=[]  Harmonics=[]  SimulateNoise=off  Profile=off  UseLocalSampling=off  EnableSwitchedLinearOptims=on  FrequencyDomain=off  UseCCode=off  RelTol=0.001  AbsTol=1e-06  MinStep=1e-09  ToWorkspace=off  RevertToSquareIcSolve=off  NumHomotopyIterations=100  PhasorMode=off  PhasorModeNumHarmonics=1  DoDC=off  ResidualTolerance=1e-09  UseLocalSolver=off  LocalSolverChoice=NE_BACKWARD_EULER_ADVANCER  LocalSolverSampleTime=0.001  DoFixedCost=off  MaxNonlinIter=3  MaxModeIter=2  ComputeImpulses=off  ImpulseIterations=2  LinearAlgebra=Sparse  EquationFormulation=NE_TIME_EF  DelaysMemoryBudget=1024  AutomaticFiltering=on  FilteringTimeConstant=0.001  PartitionStorageMethod=AS_NEEDED  PartitionMemoryBudget=1024  PartitionMethod=FAST
  World Frame : sm_lib/Frames and Transforms/World Frame
  Conn1 : PMIOPort  Side=Right
  connections:
  Mechanism Configuration/RConn1 -- Solver Configuration/RConn1 -- Conn1/RConn1 -- World Frame/RConn1
